simulink model "inverted_pendulum"  (R2016b)
settings: Solver=VariableStepAuto  StartTime=0.0  StopTime=10  RelTol=1e-3
settings Model: Creator=Quy  LastModifiedBy=Anass

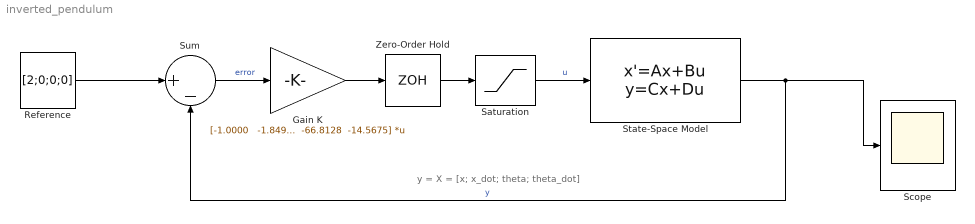
== system inverted_pendulum ==
  note: y = X = [x; x_dot; theta; theta_dot]
  "Gain K " : Gain  Gain="[-1.0000   -1.8497  -66.8128  -14.5675]"  Multiplication=Matrix(K*u) (u vector)
  Reference : Constant  Value=[2;0;0;0]
  Saturation : Saturate  UpperLimit=0.9  LowerLimit=-0.8
  Scope : Scope
  State-Space Model : StateSpace  A=|  B=|  C=eye(4)  D=[0;0;0;0]  X0=[1; 0; 0; 1]
      A=|
      | [0    1.0000         0         0;
      |          0  -10.4100         0         0;
      |          0         0         0    1.0000;
      |          0    4.3111   36.7400   -0.6249]
      B=|
      | [0;
      |    51.2860;
      |          0;
      |   -21.0230]
  Sum : Sum  Inputs=|+-
  Zero-Order Hold : ZeroOrderHold  SampleTime=0.01
  wires:
  "Gain K "/1 -> Zero-Order Hold/1
  Saturation/1 -> State-Space Model/1  "u"
  State-Space Model/1 -> Sum/2, Scope/1  "y"
  Reference/1 -> Sum/1
  Sum/1 -> "Gain K "/1  "error"
  Zero-Order Hold/1 -> Saturation/1
